simulink model "lab6"  (R2013b)
settings: Solver=ode45  StartTime=0.0  StopTime=100  RelTol=1e-3
libraries: simulink_extras x2, simulink x1, dsparch4 x1
settings Model: Creator=Kseniya  LastModifiedBy=Kseniya

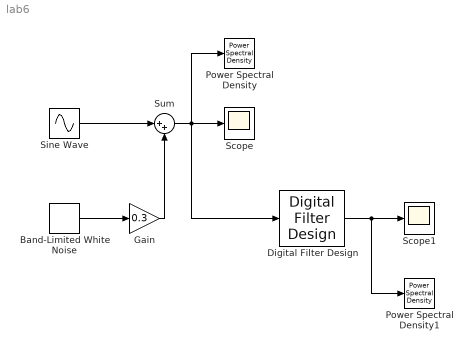
== system lab6 ==
  Band-Limited White Noise : simulink/Sources/Band-Limited White Noise  Cov=[0.3]  Ts=0.1  seed=[23341]
  Digital Filter Design : dsparch4/Digital Filter Design  mwdsp_browser_bugfix_var=off
  Gain : Gain  Gain=0.3
  Power Spectral Density : simulink_extras/Additional Sinks/Power Spectral Density  npts=128  fftpts=512  HowOften=64  sampleT=0.1
  Power Spectral Density1 : simulink_extras/Additional Sinks/Power Spectral Density  npts=128  fftpts=512  HowOften=64  sampleT=0.1
  Scope : Scope
      settings: TimeRange=40  YMin=-10  YMax=10
  Scope1 : Scope
      settings: TimeRange=40  YMin=-10  YMax=10
  Sine Wave : Sin  Amplitude=2  SampleTime=0.1
  Sum : Sum  Inputs=|++
  wires:
  Sine Wave/1 -> Sum/1
  Sum/1 -> Power Spectral Density/1, Scope/1, Digital Filter Design/1
  Digital Filter Design/1 -> Power Spectral Density1/1, Scope1/1
  Band-Limited White Noise/1 -> Gain/1
  Gain/1 -> Sum/2
